simulink model "untitled"  (R2023a)
settings: Solver=VariableStepAuto  StartTime=0.0  StopTime=10.0  RelTol=1e-3
libraries: dspfdesign x2, commrandsrc3 x1, dspsigops x1
settings Model: Creator=aa  LastModifiedBy=aa

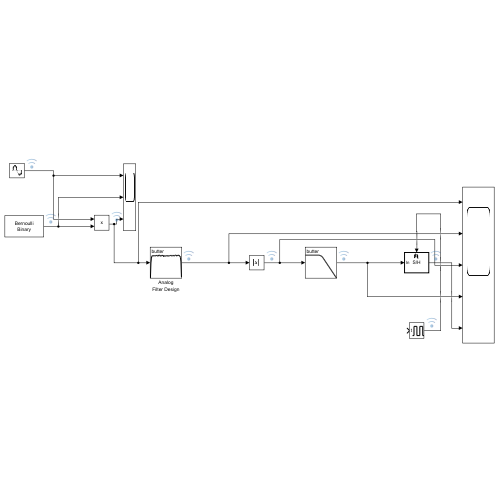
[thumbnail: Simulink's stored preview of the top-level diagram]
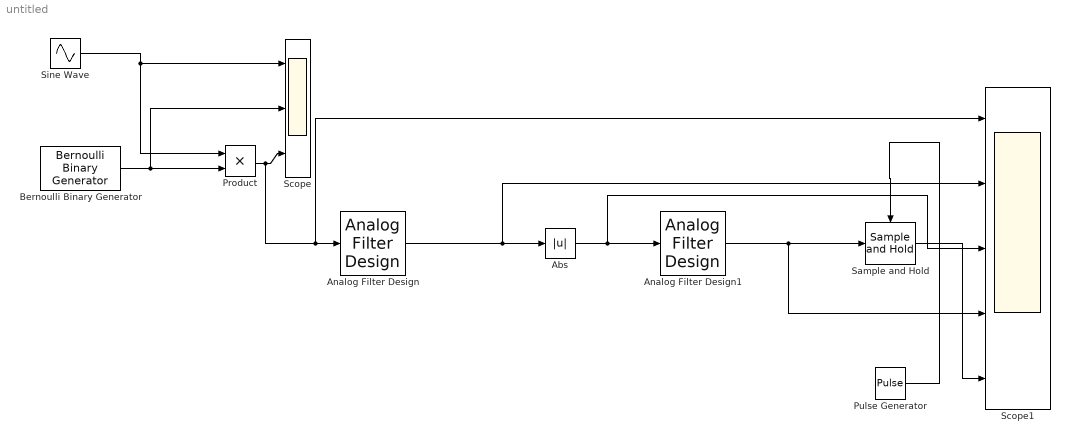
== system untitled ==
  Abs : Abs  SaturateOnIntegerOverflow=off
  Analog Filter Design : dspfdesign/Analog Filter Design  method=Butterworth  filttype=Bandpass  N=8  Wlo=0.01  Whi=50  Rp=2  Rs=40
  Analog Filter Design1 : dspfdesign/Analog Filter Design  method=Butterworth  filttype=Lowpass  N=4  Wlo=4*pi  Whi=80  Rp=2  Rs=40
  Bernoulli Binary Generator : commrandsrc3/Bernoulli Binary Generator  ProbabilityOfZero=0.5  SeedSource=Auto  Seed=0  SampleTime=1  SamplesPerFrame=1  OutputDataType=double  SimulateUsing=Interpreted execution
  Product : Product
  Pulse Generator : DiscretePulseGenerator  PulseType=Time based  TimeSource=Use external signal  PulseWidth=50
  Sample and Hold : dspsigops/Sample and Hold  trig=Either edge  initCond=0  latchinput=off
  Scope : Scope  NumInputPorts=3
  Scope1 : Scope  NumInputPorts=5
  Sine Wave : Sin  Amplitude=2  Frequency=8*pi  SampleTime=1/150
  wires:
  Sine Wave/1 -> Product/1, Scope/1
  Bernoulli Binary Generator/1 -> Scope/2, Product/2
  Analog Filter Design/1 -> Scope1/2, Abs/1
  Abs/1 -> Scope1/3, Analog Filter Design1/1
  Analog Filter Design1/1 -> Scope1/4, Sample and Hold/1
  Pulse Generator/1 -> Sample and Hold/Trigger
  Sample and Hold/1 -> Scope1/5
  Product/1 -> Scope1/1, Analog Filter Design/1, Scope/3
